simulink model "model_V1000Sim"  (R2020a)
settings: Solver=ode1  StartTime=tspan(1)  StopTime=tspan(2)  FixedStep=Ts_SimBigModel.Ts_base  RelTol=1e-3
undefined symbols (not defined in the file or in its folder): IMU1, IMU2, IMU3, mag1, mag2, SIM_SENSOR_SET
settings Model: PauseTimes=1  Creator=sl  LastModifiedBy=Administrator
settings SolverCC: AutoInsertRateTranBlk=on
settings OptimizationCC: DefaultParameterBehavior=Inlined  EnhancedBackFolding=on  PassReuseOutputArgsAs=Individual arguments  ZeroExternalMemoryAtStartup=off  ZeroInternalMemoryAtStartup=off  MaxStackSize=64  OptimizeBlockOrder=speed  DifferentSizesBufferReuse=on  OptimizationCustomize=off  EfficientTunableParamExpr=on
settings DebuggingCC: InheritedTsInSrcMsg=none  MultiTaskCondExecSysMsg=none  ParameterTunabilityLossMsg=error  UnconnectedInputMsg=none  UnconnectedOutputMsg=none  UnconnectedLineMsg=none  BusObjectLabelMismatch=error
settings HardwareCC: ProdBitPerPointer=32  ProdBitPerSizeT=32  ProdBitPerPtrDiffT=32  ProdLargestAtomicInteger=Long  ProdLargestAtomicFloat=Double  ProdWordSize=32  ProdHWDeviceType=ARM Compatible->ARM Cortex
settings ModelReferenceCC: EnableParallelModelReferenceBuilds=on  ParallelModelReferenceMATLABWorkerInit=Load Top Model
settings SFSimCC: MATLABDynamicMemAlloc=off
settings RTWCC: SystemTargetFile=ert.tlc  TemplateMakefile=ert_default_tmf  GenerateReport=on  Toolchain=GNU Tools for ARM Embedded Processors  IncludeHyperlinkInReport=on  LaunchReport=on  GenerateTraceInfo=on  GenerateTraceReport=on  GenerateTraceReportSl=on  GenerateTraceReportSf=on  GenerateTraceReportEml=on
settings CodeAppCC: ForceParamTrailComments=on  IgnoreCustomStorageClasses=off  OperatorAnnotations=on  SimulinkDataObjDesc=on  SFDataObjDesc=on  InsertBlockDesc=on
settings ERTTargetCC: InlinedParameterPlacement=NonHierarchical  ERTCustomFileTemplate=example_file_process.tlc

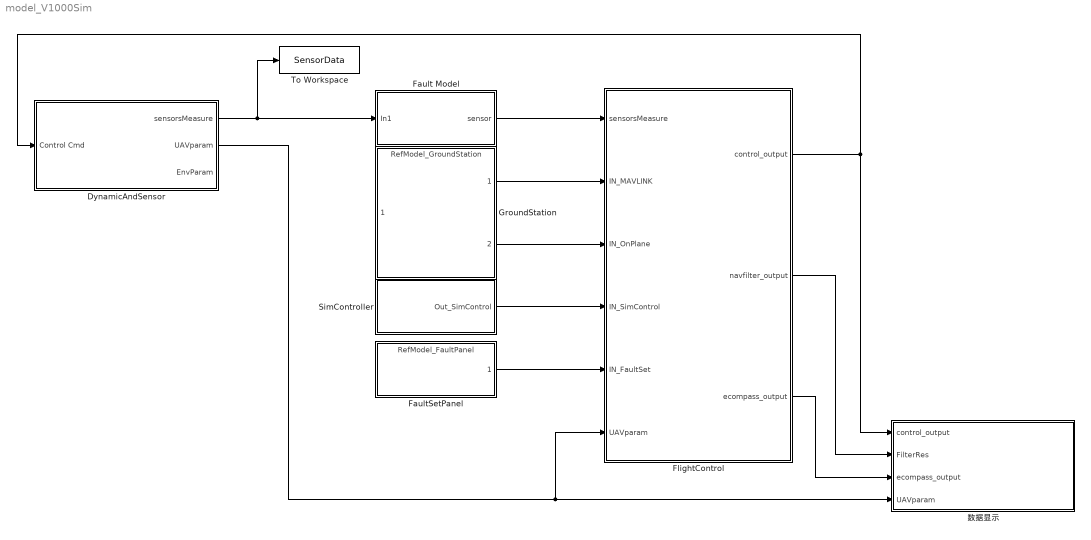
== system model_V1000Sim ==
  DynamicAndSensor : Subsystem  Variant=on
  Fault Model : Subsystem  VariantControl=SensorNoiseMode==1
  FaultSetPanel : ModelReference  ModelNameDialog=RefModel_FaultPanel  SimulationMode=Normal  ModelReferenceVersion=1.1470
  FlightControl : Subsystem
  GroundStation : ModelReference  ModelNameDialog=RefModel_GroundStation.slx  SimulationMode=Normal  CachedPortDiscreteRates=[0.04]  ModelReferenceVersion=1.3745
  SimController : Subsystem  VariantControl=SensorNoiseMode==1
  To Workspace : ToWorkspace  VariableName=SensorData  SaveFormat=Timeseries  SampleTime=-1
  数据显示 : Subsystem  Variant=on
  wires:
  FlightControl/2(navfilter_output) -> 数据显示/2(FilterRes)
  FlightControl/3(ecompass_output) -> 数据显示/3(ecompass_output)
  Fault Model/1(sensor) -> FlightControl/1(sensorsMeasure)
  DynamicAndSensor/1(sensorsMeasure) -> To Workspace/1, Fault Model/1(In1)
  DynamicAndSensor/2(UAVparam) -> FlightControl/6(UAVparam), 数据显示/4(UAVparam)
  FlightControl/1(control_output) -> DynamicAndSensor/1(Control Cmd), 数据显示/1(control_output)
  GroundStation/2 -> FlightControl/3(IN_OnPlane)
  GroundStation/1 -> FlightControl/2(IN_MAVLINK)
  SimController/1(Out_SimControl) -> FlightControl/4(IN_SimControl)
  FaultSetPanel/1 -> FlightControl/5(IN_FaultSet)

== system model_V1000Sim/DynamicAndSensor ==
  note: 1) Add Subsystem or Model blocks as valid variant choices.
      | 2) You cannot connect blocks at this level. At simulation, connectivity is automatically
      | determined, based on the active variant and port name matching.
  Control Cmd : Inport
  Flight Data : ModelReference  DisableCoverage=on  ModelNameDialog=RefModel_AeroDyn_FlightData.slx  SimulationMode=Normal  VariantControl=SimulinkRunMode == 1  ModelReferenceVersion=1.1284
  Sim Data : ModelReference  ModelNameDialog=RefModel_AeroDyn_Sim.slx  SimulationMode=Normal  VariantControl=SimulinkRunMode == 2  ModelReferenceVersion=1.1317
  sensorsMeasure : Outport
  UAVparam : Outport  Port=2
  EnvParam : Outport  Port=3  LockScale=on

== system model_V1000Sim/Fault Model ==
  In1 : Inport
  SignalFaultModel : ModelReference  Commented=through  DisableCoverage=on  ModelNameDialog=RefModel_SignalFault.slx  SimulationMode=Normal  ModelReferenceVersion=1.345
  sensor : Outport
  wires:
  In1/1 -> SignalFaultModel/1
  SignalFaultModel/1 -> sensor/1

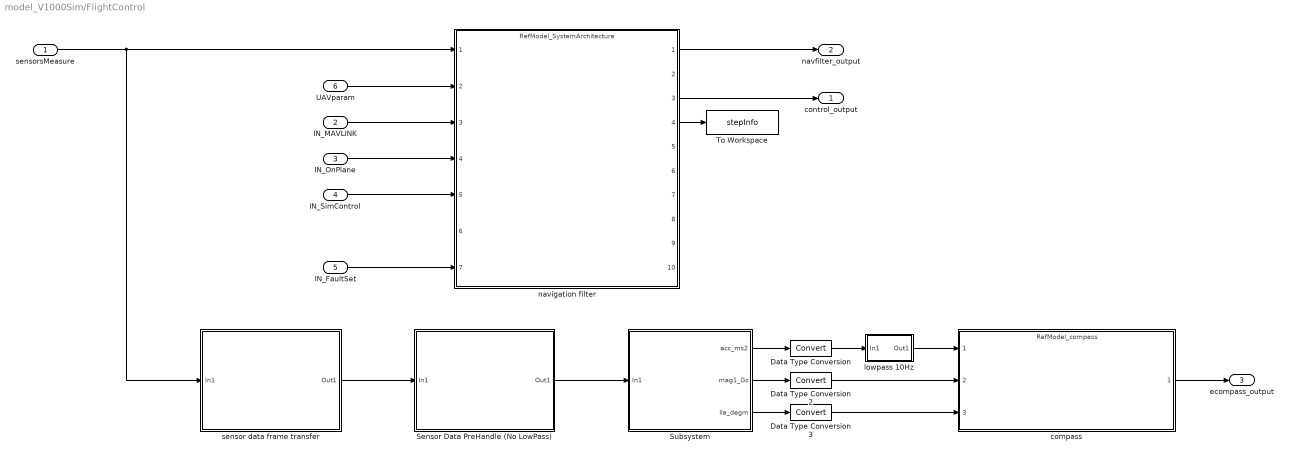
== system model_V1000Sim/FlightControl ==
  sensorsMeasure : Inport
  IN_MAVLINK : Inport  Port=2
  IN_OnPlane : Inport  Port=3
  IN_SimControl : Inport  Port=4
  IN_FaultSet : Inport  Port=5
  UAVparam : Inport  Port=6
  Data Type Conversion : DataTypeConversion
  Data Type Conversion2 : DataTypeConversion
  Data Type Conversion3 : DataTypeConversion
  Sensor Data PreHandle (No LowPass) : Subsystem
  Subsystem : Subsystem
  To Workspace : ToWorkspace  VariableName=stepInfo  SaveFormat=Timeseries  SampleTime=-1
  compass : ModelReference  ModelNameDialog=RefModel_compass.slx  SimulationMode=Normal  ModelReferenceVersion=1.16
  lowpass 10Hz : Subsystem
  navigation filter : ModelReference  ModelNameDialog=RefModel_SystemArchitecture  SimulationMode=Normal  ModelReferenceVersion=1.852
  sensor data frame transfer : Subsystem
  control_output : Outport
  navfilter_output : Outport  Port=2
  ecompass_output : Outport  Port=3
  wires:
  Subsystem/1(acc_ms2) -> Data Type Conversion/1
  Subsystem/2(mag1_Gs) -> Data Type Conversion2/1
  Subsystem/3(lla_degm) -> Data Type Conversion3/1
  Data Type Conversion2/1 -> compass/2
  Data Type Conversion3/1 -> compass/3
  Data Type Conversion/1 -> lowpass 10Hz/1(In1)
  lowpass 10Hz/1(Out1) -> compass/1
  navigation filter/1 -> navfilter_output/1
  sensorsMeasure/1 -> sensor data frame transfer/1(In1), navigation filter/1
  Sensor Data PreHandle (No LowPass)/1(Out1) -> Subsystem/1(In1)
  sensor data frame transfer/1(Out1) -> Sensor Data PreHandle (No LowPass)/1(In1)
  navigation filter/3 -> control_output/1
  UAVparam/1 -> navigation filter/2
  navigation filter/4 -> To Workspace/1
  IN_MAVLINK/1 -> navigation filter/3
  IN_OnPlane/1 -> navigation filter/4
  IN_SimControl/1 -> navigation filter/5
  compass/1 -> ecompass_output/1
  IN_FaultSet/1 -> navigation filter/7

== system model_V1000Sim/SimController ==
  10sec : Step  Time=10+33  mask(DiscretizedSource){}
      mask init:
      | %zoh
  Bus Assignment : BusAssignment  AssignedSignals=isSimOn
  Constant : Constant  Value=false
  Constant1 : Constant  Value=true
  Constant2 : Constant  Value=0  OutDataTypeStr=Bus: BUS_SIMCONTROL
  Data Type Conversion : DataTypeConversion
  Manual Switch : ManualSwitch
  Manual Switch1 : ManualSwitch
  Out_SimControl : Outport
  wires:
  Constant/1 -> Manual Switch/1
  Constant1/1 -> Manual Switch/2
  Constant2/1 -> Bus Assignment/1
  Bus Assignment/1 -> Out_SimControl/1
  Manual Switch1/1 -> Bus Assignment/2
  Manual Switch/1 -> Manual Switch1/2
  10sec/1 -> Data Type Conversion/1
  Data Type Conversion/1 -> Manual Switch1/1

== system model_V1000Sim/数据显示 ==
  note: 1) Add Subsystem or Model blocks as valid variant choices.
      | 2) You cannot connect blocks at this level. At simulation, connectivity is automatically
      | determined, based on the active variant and port name matching.
  control_output : Inport
  FilterRes : Inport  Port=2
  ecompass_output : Inport  Port=3
  UAVparam : Inport  Port=4
  Flight Data : Subsystem  VariantControl=SimulinkRunMode == 1
  Sim Data : Subsystem  VariantControl=SimulinkRunMode == 2

== system model_V1000Sim/FlightControl/Sensor Data PreHandle (No LowPass) ==
  In1 : Inport
  Bus Assignment : BusAssignment  AssignedSignals=IMU1,IMU2,IMU3,mag1,mag2
  Bus Selector : BusSelector  OutputSignals=IMU1,IMU2,IMU3
  Bus Selector1 : BusSelector  OutputSignals=mag1,mag2
  Subsystem : Subsystem
  Subsystem1 : Subsystem
  Subsystem2 : Subsystem
  Subsystem3 : Subsystem
  Subsystem4 : Subsystem
  Out1 : Outport
  wires:
  Bus Selector1/2 -> Subsystem4/1(In1)  "<mag2>"
  Bus Selector1/1 -> Subsystem3/1(In1)  "<mag1>"
  Bus Selector/3 -> Subsystem2/1(In1)  "<IMU3>"
  Bus Selector/2 -> Subsystem1/1(In1)  "<IMU2>"
  Bus Selector/1 -> Subsystem/1(In1)  "<IMU1>"
  Subsystem4/1(Out1) -> Bus Assignment/6  "mag2"
  Subsystem3/1(Out1) -> Bus Assignment/5  "mag1"
  In1/1 -> Bus Selector/1, Bus Assignment/1, Bus Selector1/1
  Bus Assignment/1 -> Out1/1
  Subsystem2/1(Out1) -> Bus Assignment/4  "IMU3"
  Subsystem1/1(Out1) -> Bus Assignment/3  "IMU2"
  Subsystem/1(Out1) -> Bus Assignment/2  "IMU1"

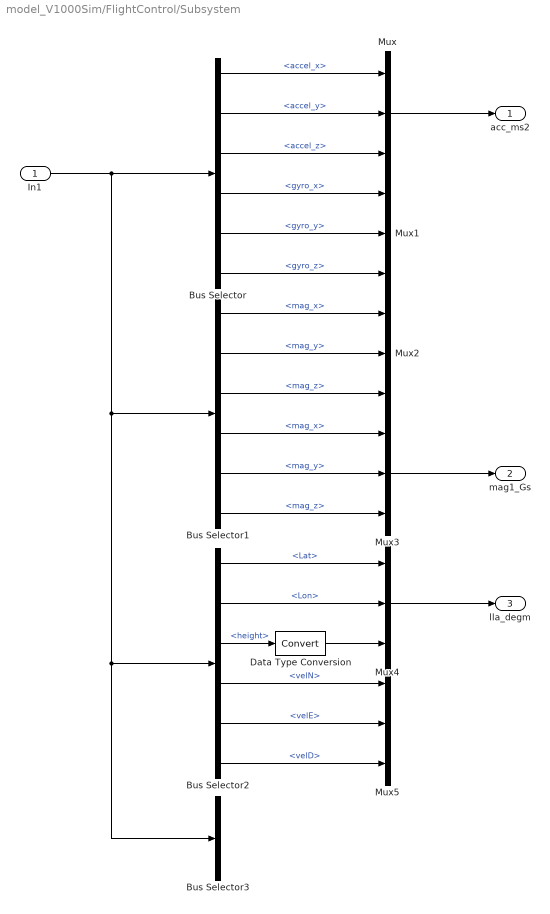
== system model_V1000Sim/FlightControl/Subsystem ==
  In1 : Inport
  Bus Selector : BusSelector  OutputSignals=IMU1.accel_x,IMU1.accel_y,IMU1.accel_z,IMU1.gyro_x,IMU1.gyro_y,IMU1.gyro_z
  Bus Selector1 : BusSelector  OutputSignals=mag1.mag_x,mag1.mag_y,mag1.mag_z,mag2.mag_x,mag2.mag_y,mag2.mag_z
  Bus Selector2 : BusSelector  OutputSignals=ublox1.Lat,ublox1.Lon,ublox1.height,ublox1.velN,ublox1.velE,ublox1.velD
  Bus Selector3 : BusSelector  OutputSignals=baro1.alt_baro,radar1.Range
  Data Type Conversion : DataTypeConversion
  Mux{,1..5} (6 alike) : Mux  Inputs=3
  acc_ms2 : Outport
  mag1_Gs : Outport  Port=2
  lla_degm : Outport  Port=3
  wires:
  In1/1 -> Bus Selector3/1, Bus Selector2/1, Bus Selector1/1, Bus Selector/1
  Bus Selector/1 -> Mux/1  "<accel_x>"
  Bus Selector/2 -> Mux/2  "<accel_y>"
  Bus Selector/3 -> Mux/3  "<accel_z>"
  Bus Selector/4 -> Mux1/1  "<gyro_x>"
  Bus Selector/5 -> Mux1/2  "<gyro_y>"
  Bus Selector/6 -> Mux1/3  "<gyro_z>"
  Mux/1 -> acc_ms2/1
  Bus Selector1/1 -> Mux2/1  "<mag_x>"
  Bus Selector1/2 -> Mux2/2  "<mag_y>"
  Bus Selector1/3 -> Mux2/3  "<mag_z>"
  Bus Selector1/4 -> Mux3/1  "<mag_x>"
  Bus Selector1/5 -> Mux3/2  "<mag_y>"
  Bus Selector1/6 -> Mux3/3  "<mag_z>"
  Bus Selector2/6 -> Mux5/3  "<velD>"
  Bus Selector2/5 -> Mux5/2  "<velE>"
  Bus Selector2/4 -> Mux5/1  "<velN>"
  Bus Selector2/3 -> Data Type Conversion/1  "<height>"
  Bus Selector2/2 -> Mux4/2  "<Lon>"
  Bus Selector2/1 -> Mux4/1  "<Lat>"
  Mux4/1 -> lla_degm/1
  Data Type Conversion/1 -> Mux4/3
  Mux3/1 -> mag1_Gs/1

== system model_V1000Sim/FlightControl/lowpass 10Hz ==
  In1 : Inport
  Demux : Demux  Outputs=3
  Mux : Mux  Inputs=3
  Mux1 : Mux  Inputs=2
  Mux2 : Mux  Inputs=2
  Mux3 : Mux  Inputs=2
  Scope : Scope  NumInputPorts=3
  Transfer Fcn : TransferFcn  Denominator=[.1 1]
  Transfer Fcn1 : TransferFcn  Denominator=[.1 1]
  Transfer Fcn2 : TransferFcn  Denominator=[.1 1]
  Out1 : Outport
  wires:
  In1/1 -> Demux/1
  Demux/1 -> Mux1/1, Transfer Fcn/1  "orignial x"
  Demux/2 -> Mux2/1, Transfer Fcn1/1  "orignial y"
  Mux/1 -> Out1/1
  Transfer Fcn1/1 -> Mux2/2, Mux/2  "filter y"
  Transfer Fcn2/1 -> Mux3/2, Mux/3  "filter z"
  Transfer Fcn/1 -> Mux1/2, Mux/1  "filter x"
  Demux/3 -> Mux3/1, Transfer Fcn2/1  "orignial z"
  Mux1/1 -> Scope/1  "ax"
  Mux2/1 -> Scope/2  "ay"
  Mux3/1 -> Scope/3  "az"

== system model_V1000Sim/FlightControl/sensor data frame transfer ==
  In1 : Inport
  Bus Assignment : BusAssignment  AssignedSignals=IMU1,IMU2,IMU3,mag1,mag2
  Bus Selector : BusSelector  OutputSignals=IMU1,IMU2,IMU3
  Bus Selector1 : BusSelector  OutputSignals=mag1,mag2
  SensorFrame to BodyFrame : Subsystem
  SensorFrame to BodyFrame1 : Subsystem
  SensorFrame to BodyFrame2 : Subsystem
  SensorFrame to BodyFrame3 : Subsystem
  SensorFrame to BodyFrame4 : Subsystem
  Out1 : Outport
  wires:
  Bus Selector/1 -> SensorFrame to BodyFrame/1(In1)  "<IMU1>"
  Bus Selector/2 -> SensorFrame to BodyFrame1/1(In1)  "<IMU2>"
  Bus Selector/3 -> SensorFrame to BodyFrame2/1(In1)  "<IMU3>"
  SensorFrame to BodyFrame/1(Out1) -> Bus Assignment/2  "IMU1"
  SensorFrame to BodyFrame1/1(Out1) -> Bus Assignment/3  "IMU2"
  SensorFrame to BodyFrame2/1(Out1) -> Bus Assignment/4  "IMU3"
  Bus Assignment/1 -> Out1/1
  In1/1 -> Bus Selector1/1, Bus Assignment/1, Bus Selector/1
  Bus Selector1/1 -> SensorFrame to BodyFrame3/1(In1)  "<mag1>"
  Bus Selector1/2 -> SensorFrame to BodyFrame4/1(In1)  "<mag2>"
  SensorFrame to BodyFrame3/1(Out1) -> Bus Assignment/5  "mag1"
  SensorFrame to BodyFrame4/1(Out1) -> Bus Assignment/6  "mag2"

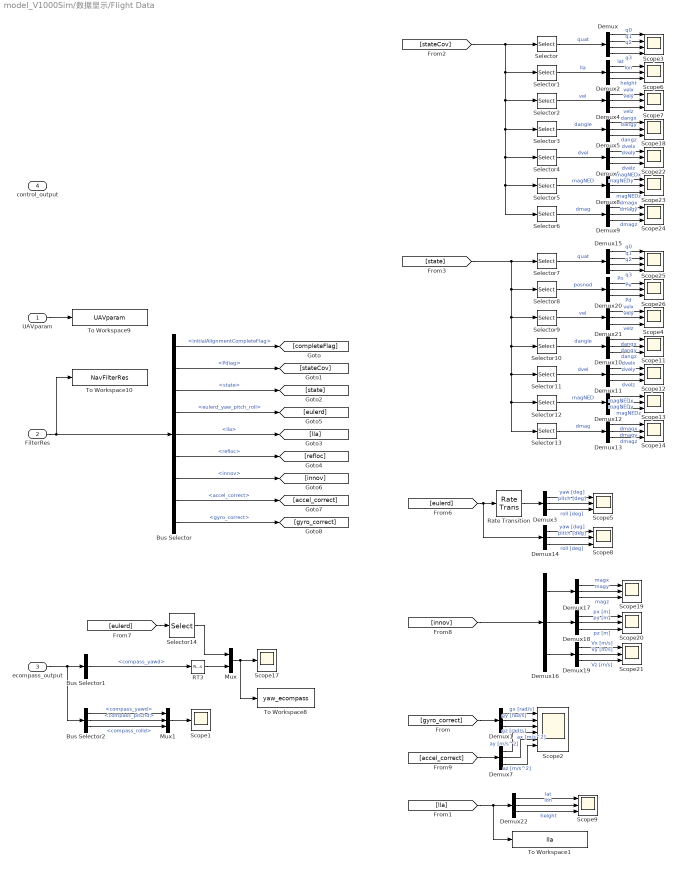
== system model_V1000Sim/数据显示/Flight Data ==
  UAVparam : Inport
  FilterRes : Inport  Port=2
  ecompass_output : Inport  Port=3
  control_output : Inport  Port=4
  Bus Selector : BusSelector  OutputSignals=initialAlignmentCompleteFlag,Pdiag,state,eulerd_yaw_pitch_roll,lla,refloc,innov,accel_correct,gyro_correct
  Bus Selector1 : BusSelector  OutputSignals=compass_yawd
  Bus Selector2 : BusSelector  OutputSignals=compass_yawd,compass_pitchd,compass_rolld
  Demux : Demux
  Demux{1..14,16..22} (21 alike) : Demux  Outputs=3
  Demux15 : Demux
  Mux : Mux  Inputs=2
  Mux1 : Mux  Inputs=3
  RT3 : RateTransition
  Rate Transition : RateTransition  OutPortSampleTime=0.012
  Scope1 : Scope
  Scope{4..9,11..14,18..24,26} (18 alike) : Scope  NumInputPorts=3
  Scope17 : Scope
  Scope2 : Scope  NumInputPorts=6
  Scope25 : Scope  NumInputPorts=4
  Scope3 : Scope  NumInputPorts=4
  Selector : Selector  InputPortWidth=nStateMARG  IndexOptions=Index vector (dialog)  Indices=[1:4]  OutputSizes=1
  Selector1 : Selector  InputPortWidth=nStateMARG  IndexOptions=Index vector (dialog)  Indices=[5:7]  OutputSizes=1
  Selector10 : Selector  InputPortWidth=nStateMARG  IndexOptions=Index vector (dialog)  Indices=[11:13]  OutputSizes=1
  Selector11 : Selector  InputPortWidth=nStateMARG  IndexOptions=Index vector (dialog)  Indices=[14:16]  OutputSizes=1
  Selector12 : Selector  InputPortWidth=nStateMARG  IndexOptions=Index vector (dialog)  Indices=[17:19]  OutputSizes=1
  Selector13 : Selector  InputPortWidth=nStateMARG  IndexOptions=Index vector (dialog)  Indices=[20:22]  OutputSizes=1
  Selector14 : Selector  InputPortWidth=3  IndexOptions=Index vector (dialog)  Indices=1  OutputSizes=1
  Selector2 : Selector  InputPortWidth=nStateMARG  IndexOptions=Index vector (dialog)  Indices=[8:10]  OutputSizes=1
  Selector3 : Selector  InputPortWidth=nStateMARG  IndexOptions=Index vector (dialog)  Indices=[11:13]  OutputSizes=1
  Selector4 : Selector  InputPortWidth=nStateMARG  IndexOptions=Index vector (dialog)  Indices=[14:16]  OutputSizes=1
  Selector5 : Selector  InputPortWidth=nStateMARG  IndexOptions=Index vector (dialog)  Indices=[17:19]  OutputSizes=1
  Selector6 : Selector  InputPortWidth=nStateMARG  IndexOptions=Index vector (dialog)  Indices=[20:22]  OutputSizes=1
  Selector7 : Selector  InputPortWidth=nStateMARG  IndexOptions=Index vector (dialog)  Indices=[1:4]  OutputSizes=1
  Selector8 : Selector  InputPortWidth=nStateMARG  IndexOptions=Index vector (dialog)  Indices=[5:7]  OutputSizes=1
  Selector9 : Selector  InputPortWidth=nStateMARG  IndexOptions=Index vector (dialog)  Indices=[8:10]  OutputSizes=1
  To Workspace1 : ToWorkspace  VariableName=lla  SaveFormat=Timeseries  SampleTime=-1
  To Workspace10 : ToWorkspace  VariableName=NavFilterRes  SaveFormat=Timeseries  SampleTime=-1
  To Workspace8 : ToWorkspace  VariableName=yaw_ecompass  SaveFormat=Timeseries  SampleTime=-1
  To Workspace9 : ToWorkspace  VariableName=UAVparam  SaveFormat=Timeseries  SampleTime=-1
  wires:
  Demux13/1 -> Scope14/1  "dmagx"
  Demux16/2 -> Demux18/1
  Demux21/3 -> Scope4/3  "velz"
  Demux12/1 -> Scope13/1  "magNEDx"
  Selector14/1 -> Mux/1
  Demux10/1 -> Scope11/1  "dangx"
  Demux12/2 -> Scope13/2  "magNEDy"
  Selector10/1 -> Demux10/1  "dangle"
  Demux15/4 -> Scope25/4  "q3"
  Demux19/2 -> Scope21/2  "Vy [m/s]"
  Selector1/1 -> Demux2/1  "lla"
  Demux3/2 -> Scope5/2  "pitch [deg]"
  Demux18/1 -> Scope20/1  "px [m]"
  [state] -> Selector8/1, Selector11/1, Selector12/1, Selector13/1, Selector10/1, Selector9/1, Selector7/1
  Demux5/2 -> Scope18/2  "dangy"
  Selector12/1 -> Demux12/1  "magNED"
  Selector13/1 -> Demux13/1  "dmag"
  Demux17/2 -> Scope19/2  "magy"
  Demux11/1 -> Scope12/1  "dvelx"
  [innov] -> Demux16/1
  Demux18/2 -> Scope20/2  "py [m]"
  Demux11/2 -> Scope12/2  "dvely"
  Demux15/3 -> Scope25/3  "q2"
  Demux16/3 -> Demux19/1
  Demux19/1 -> Scope21/1  "Vx [m/s]"
  Demux6/3 -> Scope22/3  "dvelz"
  Mux/1 -> To Workspace8/1, Scope17/1
  Demux15/2 -> Scope25/2  "q1"
  Bus Selector1/1 -> RT3/1  "<compass_yawd>"
  [eulerd] -> Demux14/1, Rate Transition/1
  [eulerd] -> Selector14/1
  Demux17/3 -> Scope19/3  "magz"
  Demux10/3 -> Scope11/3  "dangz"
  Demux21/1 -> Scope4/1  "velx"
  Demux/2 -> Scope3/2  "q1"
  Demux16/1 -> Demux17/1
  Demux/1 -> Scope3/1  "q0"
  [stateCov] -> Selector/1, Selector3/1, Selector4/1, Selector5/1, Selector6/1, Selector2/1, Selector1/1
  Demux9/2 -> Scope24/2  "dmagy"
  Demux/3 -> Scope3/3  "q2"
  Selector2/1 -> Demux4/1  "vel"
  Demux19/3 -> Scope21/3  "Vz [m/s]"
  Demux13/2 -> Scope14/2  "dmagy"
  Selector6/1 -> Demux9/1  "dmag"
  Demux17/1 -> Scope19/1  "magx"
  RT3/1 -> Mux/2
  Demux/4 -> Scope3/4  "q3"
  Demux2/1 -> Scope6/1  "lat"
  Demux2/3 -> Scope6/3  "height"
  Selector/1 -> Demux/1  "quat"
  Demux5/3 -> Scope18/3  "dangz"
  Demux4/3 -> Scope7/3  "velz"
  Demux10/2 -> Scope11/2  "dangy"
  Demux4/2 -> Scope7/2  "vely"
  Demux8/2 -> Scope23/2  "magNEDy"
  Demux18/3 -> Scope20/3  "pz [m]"
  Selector3/1 -> Demux5/1  "dangle"
  Demux2/2 -> Scope6/2  "lon"
  Selector5/1 -> Demux8/1  "magNED"
  Demux8/1 -> Scope23/1  "magNEDx"
  Demux6/2 -> Scope22/2  "dvely"
  Demux9/3 -> Scope24/3  "dmagz"
  Demux12/3 -> Scope13/3  "magNEDz"
  Demux3/3 -> Scope5/3  "roll [deg]"
  Demux21/2 -> Scope4/2  "vely"
  Demux8/3 -> Scope23/3  "magNEDz"
  Selector11/1 -> Demux11/1  "dvel"
  Selector9/1 -> Demux21/1  "vel"
  Demux20/3 -> Scope26/3  "Pd"
  Selector7/1 -> Demux15/1  "quat"
  Demux13/3 -> Scope14/3  "dmagz"
  Demux20/2 -> Scope26/2  "Pe"
  Selector4/1 -> Demux6/1  "dvel"
  Selector8/1 -> Demux20/1  "posned"
  Demux3/1 -> Scope5/1  "yaw [deg]"
  Demux11/3 -> Scope12/3  "dvelz"
  Demux15/1 -> Scope25/1  "q0"
  Demux20/1 -> Scope26/1  "Pn"
  Demux5/1 -> Scope18/1  "dangx"
  Demux6/1 -> Scope22/1  "dvelx"
  Demux4/1 -> Scope7/1  "velx"
  Demux9/1 -> Scope24/1  "dmagx"
  FilterRes/1 -> To Workspace10/1, Bus Selector/1
  Bus Selector/4 -> [eulerd]  "<eulerd_yaw_pitch_roll>"
  Bus Selector/3 -> [state]  "<state>"
  Bus Selector/5 -> [lla]  "<lla>"
  Bus Selector/2 -> [stateCov]  "<Pdiag>"
  Bus Selector/6 -> [refloc]  "<refloc>"
  Bus Selector/1 -> [completeFlag]  "<initialAlignmentCompleteFlag>"
  Bus Selector/7 -> [innov]  "<innov>"
  ecompass_output/1 -> Bus Selector2/1, Bus Selector1/1
  Bus Selector/8 -> [accel_correct]  "<accel_correct>"
  Bus Selector/9 -> [gyro_correct]  "<gyro_correct>"
  Bus Selector2/1 -> Mux1/1  "<compass_yawd>"
  Bus Selector2/2 -> Mux1/2  "<compass_pitchd>"
  Bus Selector2/3 -> Mux1/3  "<compass_rolld>"
  Mux1/1 -> Scope1/1
  [gyro_correct] -> Demux1/1
  [accel_correct] -> Demux7/1
  Demux1/1 -> Scope2/1  "gx [rad/s]"
  Demux1/2 -> Scope2/2  "gy [rad/s]"
  Demux1/3 -> Scope2/3  "gz [rad/s]"
  Demux7/1 -> Scope2/4  "ax [m/s^2]"
  Demux7/2 -> Scope2/5  "ay [m/s^2]"
  Demux7/3 -> Scope2/6  "az [m/s^2]"
  UAVparam/1 -> To Workspace9/1
  Rate Transition/1 -> Demux3/1
  Demux14/1 -> Scope8/1  "yaw [deg]"
  Demux14/3 -> Scope8/3  "roll [deg]"
  Demux14/2 -> Scope8/2  "pitch [deg]"
  Demux22/1 -> Scope9/1  "lat"
  Demux22/2 -> Scope9/2  "lon"
  Demux22/3 -> Scope9/3  "height"
  [lla] -> To Workspace1/1, Demux22/1

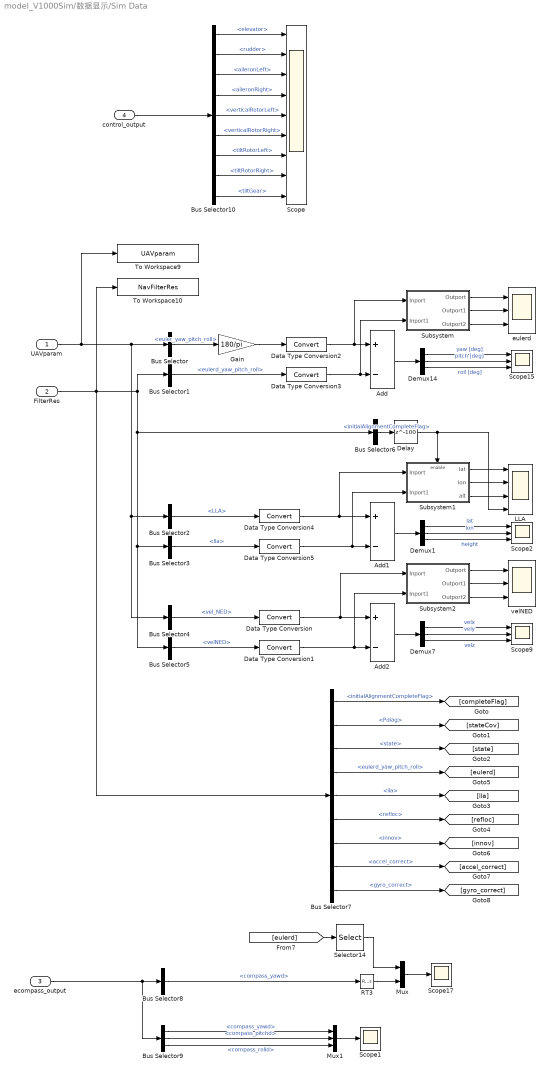
== system model_V1000Sim/数据显示/Sim Data ==
  UAVparam : Inport
  FilterRes : Inport  Port=2
  ecompass_output : Inport  Port=3
  control_output : Inport  Port=4
  Add : Sum  Inputs=+-
  Add1 : Sum  Inputs=+-
  Add2 : Sum  Inputs=+-
  Bus Selector : BusSelector  OutputSignals=euler_yaw_pitch_roll
  Bus Selector1 : BusSelector  OutputSignals=eulerd_yaw_pitch_roll
  Bus Selector10 : BusSelector  OutputSignals=elevator,rudder,aileronLeft,aileronRight,verticalRotorLeft,verticalRotorRight,tiltRotorLeft,tiltRotorRight,tiltGear
  Bus Selector2 : BusSelector  OutputSignals=LLA
  Bus Selector3 : BusSelector  OutputSignals=lla
  Bus Selector4 : BusSelector  OutputSignals=vel_NED
  Bus Selector5 : BusSelector  OutputSignals=velNED
  Bus Selector6 : BusSelector  OutputSignals=initialAlignmentCompleteFlag
  Bus Selector7 : BusSelector  OutputSignals=initialAlignmentCompleteFlag,Pdiag,state,eulerd_yaw_pitch_roll,lla,refloc,innov,accel_correct,gyro_correct
  Bus Selector8 : BusSelector  OutputSignals=compass_yawd
  Bus Selector9 : BusSelector  OutputSignals=compass_yawd,compass_pitchd,compass_rolld
  Data Type Conversion{,1..5} (6 alike) : DataTypeConversion
  Delay : Delay  DelayLength=100
  Demux1 : Demux  Outputs=3
  Demux14 : Demux  Outputs=3
  Demux7 : Demux  Outputs=3
  Gain : Gain  Gain=180/pi
  LLA : Scope  NumInputPorts=4
  Mux : Mux  Inputs=2
  Mux1 : Mux  Inputs=3
  RT3 : RateTransition
  Scope : Scope  NumInputPorts=9
  Scope1 : Scope
  Scope15 : Scope  NumInputPorts=3
  Scope17 : Scope
  Scope2 : Scope  NumInputPorts=3
  Scope9 : Scope  NumInputPorts=3
  Selector14 : Selector  InputPortWidth=3  IndexOptions=Index vector (dialog)  Indices=1  OutputSizes=1
  Subsystem : Subsystem
  Subsystem1 : Subsystem
  Subsystem2 : Subsystem
  To Workspace10 : ToWorkspace  VariableName=NavFilterRes  SaveFormat=Timeseries  SampleTime=-1
  To Workspace9 : ToWorkspace  VariableName=UAVparam  SaveFormat=Timeseries  SampleTime=-1
  eulerd : Scope  NumInputPorts=3
  velNED : Scope  NumInputPorts=3
  wires:
  Demux14/3 -> Scope15/3  "roll [deg]"
  Bus Selector4/1 -> Data Type Conversion/1  "<vel_NED>"
  Demux14/2 -> Scope15/2  "pitch [deg]"
  Bus Selector2/1 -> Data Type Conversion4/1  "<LLA>"
  Demux1/3 -> Scope2/3  "height"
  Gain/1 -> Data Type Conversion2/1
  Bus Selector3/1 -> Data Type Conversion5/1  "<lla>"
  Demux1/1 -> Scope2/1  "lat"
  Demux7/3 -> Scope9/3  "velz"
  Subsystem2/3(Outport2) -> velNED/3
  Bus Selector1/1 -> Data Type Conversion3/1  "<eulerd_yaw_pitch_roll>"
  Subsystem2/2(Outport1) -> velNED/2
  Demux7/1 -> Scope9/1  "velx"
  Demux14/1 -> Scope15/1  "yaw [deg]"
  Subsystem1/2(lon) -> LLA/2
  Add2/1 -> Demux7/1
  Add1/1 -> Demux1/1
  Subsystem1/1(lat) -> LLA/1
  Subsystem/3(Outport2) -> eulerd/3
  Demux1/2 -> Scope2/2  "lon"
  Add/1 -> Demux14/1
  Subsystem2/1(Outport) -> velNED/1
  Bus Selector/1 -> Gain/1  "<euler_yaw_pitch_roll>"
  Demux7/2 -> Scope9/2  "vely"
  Subsystem1/3(alt) -> LLA/3
  Subsystem/2(Outport1) -> eulerd/2
  Subsystem/1(Outport) -> eulerd/1
  Bus Selector5/1 -> Data Type Conversion1/1  "<velNED>"
  UAVparam/1 -> To Workspace9/1, Bus Selector2/1, Bus Selector4/1, Bus Selector/1
  Bus Selector6/1 -> Delay/1  "<initialAlignmentCompleteFlag>"
  Delay/1 -> LLA/4, Subsystem1/Enable
  FilterRes/1 -> Bus Selector7/1, Bus Selector6/1, Bus Selector3/1, Bus Selector5/1, Bus Selector1/1, To Workspace10/1
  Mux1/1 -> Scope1/1
  Bus Selector9/3 -> Mux1/3  "<compass_rolld>"
  Bus Selector9/1 -> Mux1/1  "<compass_yawd>"
  Bus Selector9/2 -> Mux1/2  "<compass_pitchd>"
  [eulerd] -> Selector14/1
  Mux/1 -> Scope17/1
  Bus Selector8/1 -> RT3/1  "<compass_yawd>"
  RT3/1 -> Mux/2
  ecompass_output/1 -> Bus Selector9/1, Bus Selector8/1
  Selector14/1 -> Mux/1
  Bus Selector7/8 -> [accel_correct]  "<accel_correct>"
  Bus Selector7/3 -> [state]  "<state>"
  Bus Selector7/9 -> [gyro_correct]  "<gyro_correct>"
  Bus Selector7/7 -> [innov]  "<innov>"
  Bus Selector7/2 -> [stateCov]  "<Pdiag>"
  Bus Selector7/6 -> [refloc]  "<refloc>"
  Bus Selector7/1 -> [completeFlag]  "<initialAlignmentCompleteFlag>"
  Bus Selector7/5 -> [lla]  "<lla>"
  Bus Selector7/4 -> [eulerd]  "<eulerd_yaw_pitch_roll>"
  Data Type Conversion/1 -> Subsystem2/1(Inport), Add2/1
  Data Type Conversion1/1 -> Subsystem2/2(Inport1), Add2/2
  Data Type Conversion2/1 -> Subsystem/1(Inport), Add/1
  Data Type Conversion3/1 -> Subsystem/2(Inport1), Add/2
  Data Type Conversion4/1 -> Subsystem1/1(Inport), Add1/1
  Data Type Conversion5/1 -> Subsystem1/2(Inport1), Add1/2
  Bus Selector10/8 -> Scope/8  "<tiltRotorRight>"
  Bus Selector10/6 -> Scope/6  "<verticalRotorRight>"
  Bus Selector10/1 -> Scope/1  "<elevator>"
  Bus Selector10/7 -> Scope/7  "<tiltRotorLeft>"
  Bus Selector10/2 -> Scope/2  "<rudder>"
  Bus Selector10/5 -> Scope/5  "<verticalRotorLeft>"
  Bus Selector10/3 -> Scope/3  "<aileronLeft>"
  Bus Selector10/4 -> Scope/4  "<aileronRight>"
  Bus Selector10/9 -> Scope/9  "<tiltGear>"
  control_output/1 -> Bus Selector10/1

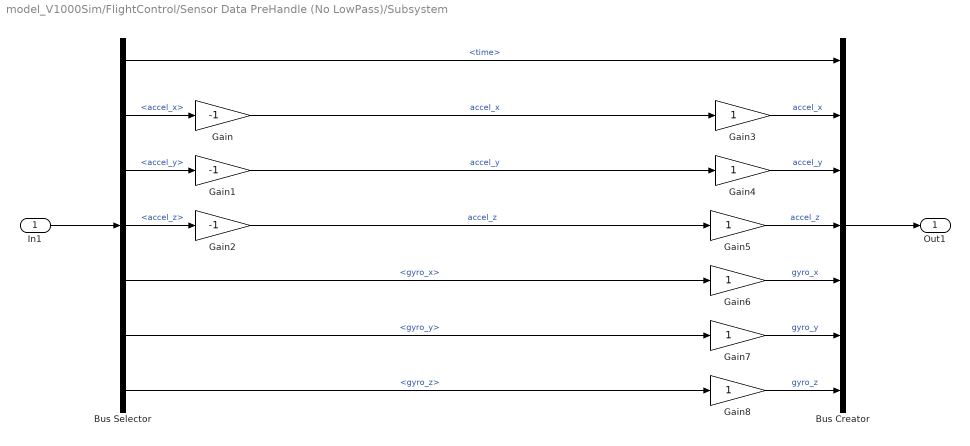
== system model_V1000Sim/FlightControl/Sensor Data PreHandle (No LowPass)/Subsystem ==
  In1 : Inport
  Bus Creator : BusCreator  Inputs=7
  Bus Selector : BusSelector  OutputSignals=time,accel_x,accel_y,accel_z,gyro_x,gyro_y,gyro_z
  Gain : Gain  Gain=-1
  Gain1 : Gain  Gain=-1
  Gain2 : Gain  Gain=-1
  Gain{3..8} (6 alike) : Gain
  Out1 : Outport
  wires:
  Gain8/1 -> Bus Creator/7  "gyro_z"
  Gain7/1 -> Bus Creator/6  "gyro_y"
  Gain6/1 -> Bus Creator/5  "gyro_x"
  Gain5/1 -> Bus Creator/4  "accel_z"
  Gain4/1 -> Bus Creator/3  "accel_y"
  Gain3/1 -> Bus Creator/2  "accel_x"
  Bus Selector/7 -> Gain8/1  "<gyro_z>"
  Bus Selector/6 -> Gain7/1  "<gyro_y>"
  Bus Selector/5 -> Gain6/1  "<gyro_x>"
  Gain2/1 -> Gain5/1  "accel_z"
  Gain1/1 -> Gain4/1  "accel_y"
  Gain/1 -> Gain3/1  "accel_x"
  Bus Selector/1 -> Bus Creator/1  "<time>"
  Bus Selector/4 -> Gain2/1  "<accel_z>"
  Bus Selector/3 -> Gain1/1  "<accel_y>"
  Bus Selector/2 -> Gain/1  "<accel_x>"
  Bus Creator/1 -> Out1/1
  In1/1 -> Bus Selector/1

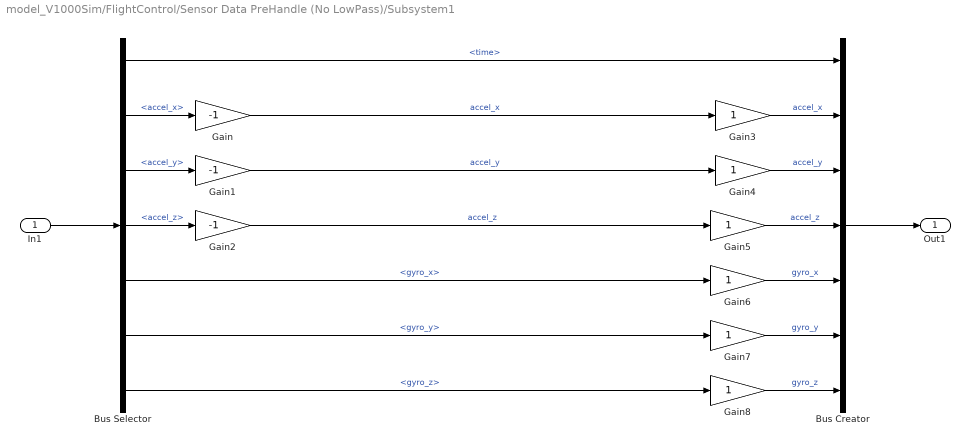
== system model_V1000Sim/FlightControl/Sensor Data PreHandle (No LowPass)/Subsystem1 ==
  In1 : Inport
  Bus Creator : BusCreator  Inputs=7
  Bus Selector : BusSelector  OutputSignals=time,accel_x,accel_y,accel_z,gyro_x,gyro_y,gyro_z
  Gain : Gain  Gain=-1
  Gain1 : Gain  Gain=-1
  Gain2 : Gain  Gain=-1
  Gain{3..8} (6 alike) : Gain
  Out1 : Outport
  wires:
  In1/1 -> Bus Selector/1
  Bus Creator/1 -> Out1/1
  Bus Selector/2 -> Gain/1  "<accel_x>"
  Bus Selector/3 -> Gain1/1  "<accel_y>"
  Bus Selector/4 -> Gain2/1  "<accel_z>"
  Bus Selector/1 -> Bus Creator/1  "<time>"
  Gain/1 -> Gain3/1  "accel_x"
  Gain1/1 -> Gain4/1  "accel_y"
  Gain2/1 -> Gain5/1  "accel_z"
  Bus Selector/5 -> Gain6/1  "<gyro_x>"
  Bus Selector/6 -> Gain7/1  "<gyro_y>"
  Bus Selector/7 -> Gain8/1  "<gyro_z>"
  Gain3/1 -> Bus Creator/2  "accel_x"
  Gain4/1 -> Bus Creator/3  "accel_y"
  Gain5/1 -> Bus Creator/4  "accel_z"
  Gain6/1 -> Bus Creator/5  "gyro_x"
  Gain7/1 -> Bus Creator/6  "gyro_y"
  Gain8/1 -> Bus Creator/7  "gyro_z"

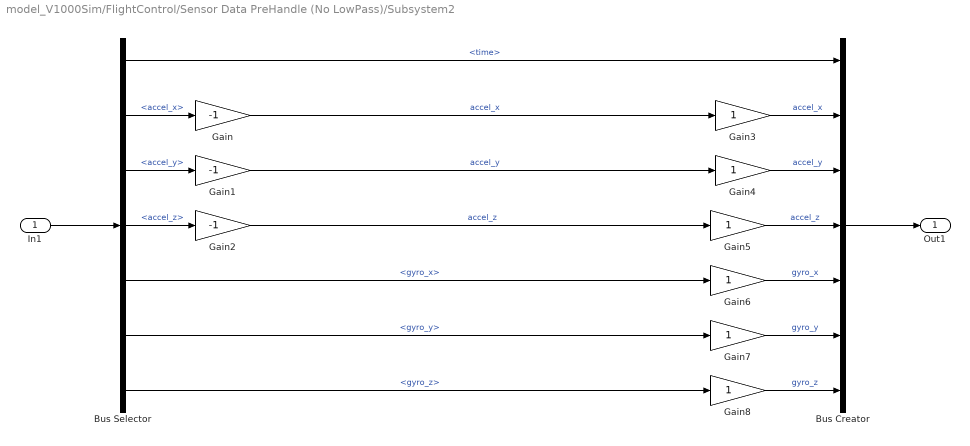
== system model_V1000Sim/FlightControl/Sensor Data PreHandle (No LowPass)/Subsystem2 ==
  In1 : Inport
  Bus Creator : BusCreator  Inputs=7
  Bus Selector : BusSelector  OutputSignals=time,accel_x,accel_y,accel_z,gyro_x,gyro_y,gyro_z
  Gain : Gain  Gain=-1
  Gain1 : Gain  Gain=-1
  Gain2 : Gain  Gain=-1
  Gain{3..8} (6 alike) : Gain
  Out1 : Outport
  wires:
  Gain8/1 -> Bus Creator/7  "gyro_z"
  Gain7/1 -> Bus Creator/6  "gyro_y"
  Gain6/1 -> Bus Creator/5  "gyro_x"
  Gain5/1 -> Bus Creator/4  "accel_z"
  Gain4/1 -> Bus Creator/3  "accel_y"
  Gain3/1 -> Bus Creator/2  "accel_x"
  Bus Selector/7 -> Gain8/1  "<gyro_z>"
  Bus Selector/6 -> Gain7/1  "<gyro_y>"
  Bus Selector/5 -> Gain6/1  "<gyro_x>"
  Gain2/1 -> Gain5/1  "accel_z"
  Gain1/1 -> Gain4/1  "accel_y"
  Gain/1 -> Gain3/1  "accel_x"
  Bus Selector/1 -> Bus Creator/1  "<time>"
  Bus Selector/4 -> Gain2/1  "<accel_z>"
  Bus Selector/3 -> Gain1/1  "<accel_y>"
  Bus Selector/2 -> Gain/1  "<accel_x>"
  Bus Creator/1 -> Out1/1
  In1/1 -> Bus Selector/1

== system model_V1000Sim/FlightControl/Sensor Data PreHandle (No LowPass)/Subsystem3 ==
  In1 : Inport
  Bus Creator : BusCreator  Inputs=4
  Bus Selector : BusSelector  OutputSignals=time,mag_x,mag_y,mag_z
  Gs to uT1 : Gain  Gain=100
  Gs to uT2 : Gain  Gain=100
  Gs to uT3 : Gain  Gain=100
  Out1 : Outport
  wires:
  Bus Selector/4 -> Gs to uT3/1  "<mag_z>"
  Bus Selector/3 -> Gs to uT2/1  "<mag_y>"
  Bus Selector/2 -> Gs to uT1/1  "<mag_x>"
  Gs to uT3/1 -> Bus Creator/4  "mag_z"
  Gs to uT2/1 -> Bus Creator/3  "mag_y"
  Gs to uT1/1 -> Bus Creator/2  "mag_x"
  In1/1 -> Bus Selector/1
  Bus Creator/1 -> Out1/1
  Bus Selector/1 -> Bus Creator/1  "<time>"

== system model_V1000Sim/FlightControl/Sensor Data PreHandle (No LowPass)/Subsystem4 ==
  In1 : Inport
  Bus Creator : BusCreator  Inputs=4
  Bus Selector : BusSelector  OutputSignals=time,mag_x,mag_y,mag_z
  Gs to uT1 : Gain  Gain=100
  Gs to uT2 : Gain  Gain=100
  Gs to uT3 : Gain  Gain=100
  Out1 : Outport
  wires:
  Bus Selector/1 -> Bus Creator/1  "<time>"
  Bus Creator/1 -> Out1/1
  In1/1 -> Bus Selector/1
  Gs to uT1/1 -> Bus Creator/2  "mag_x"
  Gs to uT2/1 -> Bus Creator/3  "mag_y"
  Gs to uT3/1 -> Bus Creator/4  "mag_z"
  Bus Selector/2 -> Gs to uT1/1  "<mag_x>"
  Bus Selector/3 -> Gs to uT2/1  "<mag_y>"
  Bus Selector/4 -> Gs to uT3/1  "<mag_z>"

== system model_V1000Sim/FlightControl/sensor data frame transfer/SensorFrame to BodyFrame ==
  In1 : Inport
  Bus Creator : BusCreator  Inputs=7
  Bus Selector : BusSelector  OutputSignals=time,accel_x,accel_y,accel_z,gyro_x,gyro_y,gyro_z
  Frame Transfer : Subsystem
  Frame Transfer1 : Subsystem
  Out1 : Outport
  wires:
  Bus Selector/1 -> Bus Creator/1  "<time>"
  Bus Creator/1 -> Out1/1
  In1/1 -> Bus Selector/1
  Bus Selector/2 -> Frame Transfer/1(In1)  "<accel_x>"
  Bus Selector/3 -> Frame Transfer/2(In2)  "<accel_y>"
  Bus Selector/4 -> Frame Transfer/3(In3)  "<accel_z>"
  Frame Transfer/1(Out1) -> Bus Creator/2  "accel_x"
  Frame Transfer/2(Out2) -> Bus Creator/3  "accel_y"
  Frame Transfer/3(Out3) -> Bus Creator/4  "accel_z"
  Bus Selector/5 -> Frame Transfer1/1(In1)  "<gyro_x>"
  Bus Selector/6 -> Frame Transfer1/2(In2)  "<gyro_y>"
  Bus Selector/7 -> Frame Transfer1/3(In3)  "<gyro_z>"
  Frame Transfer1/1(Out1) -> Bus Creator/5  "gyro_x"
  Frame Transfer1/2(Out2) -> Bus Creator/6  "gyro_y"
  Frame Transfer1/3(Out3) -> Bus Creator/7  "gyro_z"

== system model_V1000Sim/FlightControl/sensor data frame transfer/SensorFrame to BodyFrame1 ==
  In1 : Inport
  Bus Creator : BusCreator  Inputs=7
  Bus Selector : BusSelector  OutputSignals=time,accel_x,accel_y,accel_z,gyro_x,gyro_y,gyro_z
  Frame Transfer : Subsystem
  Frame Transfer1 : Subsystem
  Out1 : Outport
  wires:
  Frame Transfer1/3(Out3) -> Bus Creator/7  "gyro_z"
  Frame Transfer1/2(Out2) -> Bus Creator/6  "gyro_y"
  Frame Transfer1/1(Out1) -> Bus Creator/5  "gyro_x"
  Bus Selector/7 -> Frame Transfer1/3(In3)  "<gyro_z>"
  Bus Selector/6 -> Frame Transfer1/2(In2)  "<gyro_y>"
  Bus Selector/5 -> Frame Transfer1/1(In1)  "<gyro_x>"
  Frame Transfer/3(Out3) -> Bus Creator/4  "accel_z"
  Frame Transfer/2(Out2) -> Bus Creator/3  "accel_y"
  Frame Transfer/1(Out1) -> Bus Creator/2  "accel_x"
  Bus Selector/4 -> Frame Transfer/3(In3)  "<accel_z>"
  Bus Selector/3 -> Frame Transfer/2(In2)  "<accel_y>"
  Bus Selector/2 -> Frame Transfer/1(In1)  "<accel_x>"
  In1/1 -> Bus Selector/1
  Bus Creator/1 -> Out1/1
  Bus Selector/1 -> Bus Creator/1  "<time>"

== system model_V1000Sim/FlightControl/sensor data frame transfer/SensorFrame to BodyFrame2 ==
  In1 : Inport
  Bus Creator : BusCreator  Inputs=7
  Bus Selector : BusSelector  OutputSignals=time,accel_x,accel_y,accel_z,gyro_x,gyro_y,gyro_z
  Frame Transfer : Subsystem
  Frame Transfer1 : Subsystem
  Out1 : Outport
  wires:
  Bus Selector/1 -> Bus Creator/1  "<time>"
  Bus Creator/1 -> Out1/1
  In1/1 -> Bus Selector/1
  Bus Selector/2 -> Frame Transfer/1(In1)  "<accel_x>"
  Bus Selector/3 -> Frame Transfer/2(In2)  "<accel_y>"
  Bus Selector/4 -> Frame Transfer/3(In3)  "<accel_z>"
  Frame Transfer/1(Out1) -> Bus Creator/2  "accel_x"
  Frame Transfer/2(Out2) -> Bus Creator/3  "accel_y"
  Frame Transfer/3(Out3) -> Bus Creator/4  "accel_z"
  Bus Selector/5 -> Frame Transfer1/1(In1)  "<gyro_x>"
  Bus Selector/6 -> Frame Transfer1/2(In2)  "<gyro_y>"
  Bus Selector/7 -> Frame Transfer1/3(In3)  "<gyro_z>"
  Frame Transfer1/1(Out1) -> Bus Creator/5  "gyro_x"
  Frame Transfer1/2(Out2) -> Bus Creator/6  "gyro_y"
  Frame Transfer1/3(Out3) -> Bus Creator/7  "gyro_z"

== system model_V1000Sim/FlightControl/sensor data frame transfer/SensorFrame to BodyFrame3 ==
  In1 : Inport
  Bus Creator : BusCreator  Inputs=4
  Bus Selector : BusSelector  OutputSignals=time,mag_x,mag_y,mag_z
  Frame Transfer : Subsystem
  Out1 : Outport
  wires:
  Frame Transfer/3(Out3) -> Bus Creator/4  "mag_z"
  Frame Transfer/2(Out2) -> Bus Creator/3  "mag_y"
  Frame Transfer/1(Out1) -> Bus Creator/2  "mag_x"
  Bus Selector/4 -> Frame Transfer/3(In3)  "<mag_z>"
  Bus Selector/3 -> Frame Transfer/2(In2)  "<mag_y>"
  Bus Selector/2 -> Frame Transfer/1(In1)  "<mag_x>"
  In1/1 -> Bus Selector/1
  Bus Creator/1 -> Out1/1
  Bus Selector/1 -> Bus Creator/1  "<time>"

== system model_V1000Sim/FlightControl/sensor data frame transfer/SensorFrame to BodyFrame4 ==
  In1 : Inport
  Bus Creator : BusCreator  Inputs=4
  Bus Selector : BusSelector  OutputSignals=time,mag_x,mag_y,mag_z
  Frame Transfer : Subsystem
  Out1 : Outport
  wires:
  Bus Selector/1 -> Bus Creator/1  "<time>"
  Bus Creator/1 -> Out1/1
  In1/1 -> Bus Selector/1
  Bus Selector/2 -> Frame Transfer/1(In1)  "<mag_x>"
  Bus Selector/3 -> Frame Transfer/2(In2)  "<mag_y>"
  Bus Selector/4 -> Frame Transfer/3(In3)  "<mag_z>"
  Frame Transfer/1(Out1) -> Bus Creator/2  "mag_x"
  Frame Transfer/2(Out2) -> Bus Creator/3  "mag_y"
  Frame Transfer/3(Out3) -> Bus Creator/4  "mag_z"

== system model_V1000Sim/数据显示/Sim Data/Subsystem ==
  Inport : Inport
  Inport1 : Inport  Port=2
  Demux7 : Demux  Outputs=3
  Demux8 : Demux  Outputs=3
  Mux : Mux  Inputs=2
  Mux1 : Mux  Inputs=2
  Mux2 : Mux  Inputs=2
  Outport : Outport
  Outport1 : Outport  Port=2
  Outport2 : Outport  Port=3
  wires:
  Demux7/1 -> Mux/1  "yaw [deg]"
  Demux8/1 -> Mux/2  "yaw [deg]"
  Inport/1 -> Demux7/1
  Mux/1 -> Outport/1
  Demux8/3 -> Mux2/2  "roll [deg]"
  Demux7/2 -> Mux1/1
  Inport1/1 -> Demux8/1
  Mux2/1 -> Outport2/1
  Mux1/1 -> Outport1/1
  Demux8/2 -> Mux1/2  "pitch [deg]"
  Demux7/3 -> Mux2/1  "roll [deg]"

== system model_V1000Sim/数据显示/Sim Data/Subsystem1 ==
  Inport : Inport
  Inport1 : Inport  Port=2
  Enable : EnablePort
  Demux7 : Demux  Outputs=3
  Demux8 : Demux  Outputs=3
  Mux : Mux  Inputs=2
  Mux1 : Mux  Inputs=2
  Mux2 : Mux  Inputs=2
  lat : Outport
  lon : Outport  Port=2
  alt : Outport  Port=3
  wires:
  Demux7/3 -> Mux2/1  "roll [deg]"
  Demux8/2 -> Mux1/2  "pitch [deg]"
  Mux2/1 -> alt/1
  Inport1/1 -> Demux8/1
  Demux7/2 -> Mux1/1
  Demux8/3 -> Mux2/2  "roll [deg]"
  Inport/1 -> Demux7/1
  Demux8/1 -> Mux/2  "yaw [deg]"
  Demux7/1 -> Mux/1  "yaw [deg]"
  Mux/1 -> lat/1
  Mux1/1 -> lon/1

== system model_V1000Sim/数据显示/Sim Data/Subsystem2 ==
  Inport : Inport
  Inport1 : Inport  Port=2
  Demux7 : Demux  Outputs=3
  Demux8 : Demux  Outputs=3
  Mux : Mux  Inputs=2
  Mux1 : Mux  Inputs=2
  Mux2 : Mux  Inputs=2
  Outport : Outport
  Outport1 : Outport  Port=2
  Outport2 : Outport  Port=3
  wires:
  Demux7/1 -> Mux/1  "yaw [deg]"
  Demux8/1 -> Mux/2  "yaw [deg]"
  Inport/1 -> Demux7/1
  Mux/1 -> Outport/1
  Demux8/3 -> Mux2/2  "roll [deg]"
  Demux7/2 -> Mux1/1
  Inport1/1 -> Demux8/1
  Mux2/1 -> Outport2/1
  Mux1/1 -> Outport1/1
  Demux8/2 -> Mux1/2  "pitch [deg]"
  Demux7/3 -> Mux2/1  "roll [deg]"

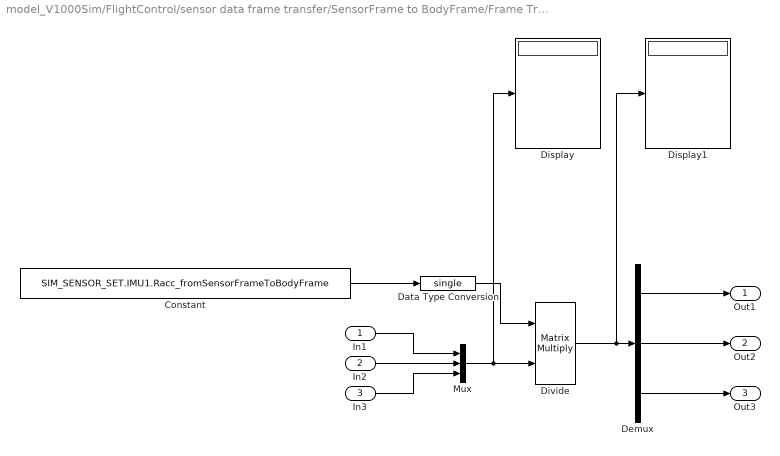
== system model_V1000Sim/FlightControl/sensor data frame transfer/SensorFrame to BodyFrame/Frame Transfer ==
  In1 : Inport
  In2 : Inport  Port=2
  In3 : Inport  Port=3
  Constant : Constant  Value=SIM_SENSOR_SET.IMU1.Racc_fromSensorFrameToBodyFrame
  Data Type Conversion : DataTypeConversion  OutDataTypeStr=single
  Demux : Demux  Outputs=3
  Display : Display
  Display1 : Display
  Divide : Product  Inputs=**  Multiplication=Matrix(*)
  Mux : Mux  Inputs=3
  Out1 : Outport
  Out2 : Outport  Port=2
  Out3 : Outport  Port=3
  wires:
  In2/1 -> Mux/2
  In1/1 -> Mux/1
  In3/1 -> Mux/3
  Constant/1 -> Data Type Conversion/1
  Mux/1 -> Display/1, Divide/2
  Divide/1 -> Display1/1, Demux/1
  Demux/1 -> Out1/1
  Demux/2 -> Out2/1
  Demux/3 -> Out3/1
  Data Type Conversion/1 -> Divide/1

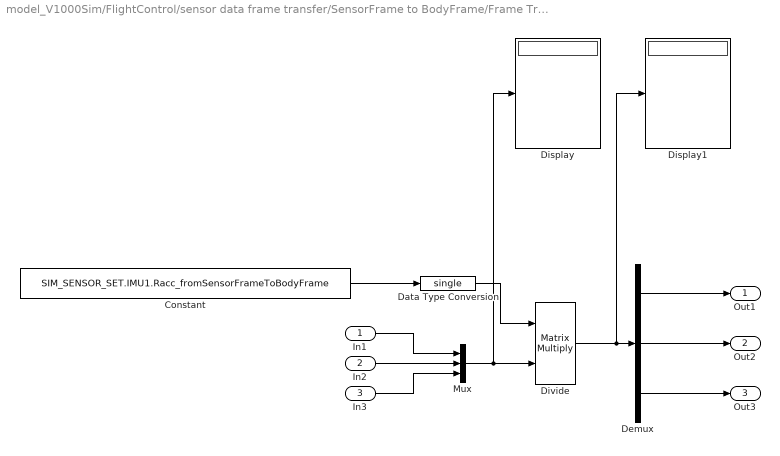
== system model_V1000Sim/FlightControl/sensor data frame transfer/SensorFrame to BodyFrame/Frame Transfer1 ==
  In1 : Inport
  In2 : Inport  Port=2
  In3 : Inport  Port=3
  Constant : Constant  Value=SIM_SENSOR_SET.IMU1.Racc_fromSensorFrameToBodyFrame
  Data Type Conversion : DataTypeConversion  OutDataTypeStr=single
  Demux : Demux  Outputs=3
  Display : Display
  Display1 : Display
  Divide : Product  Inputs=**  Multiplication=Matrix(*)
  Mux : Mux  Inputs=3
  Out1 : Outport
  Out2 : Outport  Port=2
  Out3 : Outport  Port=3
  wires:
  Data Type Conversion/1 -> Divide/1
  Demux/3 -> Out3/1
  Demux/2 -> Out2/1
  Demux/1 -> Out1/1
  Divide/1 -> Demux/1, Display1/1
  Mux/1 -> Divide/2, Display/1
  Constant/1 -> Data Type Conversion/1
  In3/1 -> Mux/3
  In1/1 -> Mux/1
  In2/1 -> Mux/2

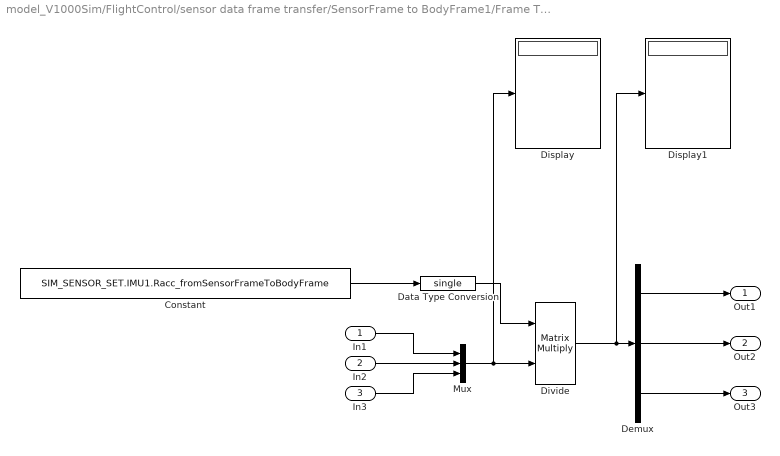
== system model_V1000Sim/FlightControl/sensor data frame transfer/SensorFrame to BodyFrame1/Frame Transfer ==
  In1 : Inport
  In2 : Inport  Port=2
  In3 : Inport  Port=3
  Constant : Constant  Value=SIM_SENSOR_SET.IMU1.Racc_fromSensorFrameToBodyFrame
  Data Type Conversion : DataTypeConversion  OutDataTypeStr=single
  Demux : Demux  Outputs=3
  Display : Display
  Display1 : Display
  Divide : Product  Inputs=**  Multiplication=Matrix(*)
  Mux : Mux  Inputs=3
  Out1 : Outport
  Out2 : Outport  Port=2
  Out3 : Outport  Port=3
  wires:
  Data Type Conversion/1 -> Divide/1
  Demux/3 -> Out3/1
  Demux/2 -> Out2/1
  Demux/1 -> Out1/1
  Divide/1 -> Demux/1, Display1/1
  Mux/1 -> Divide/2, Display/1
  Constant/1 -> Data Type Conversion/1
  In3/1 -> Mux/3
  In1/1 -> Mux/1
  In2/1 -> Mux/2

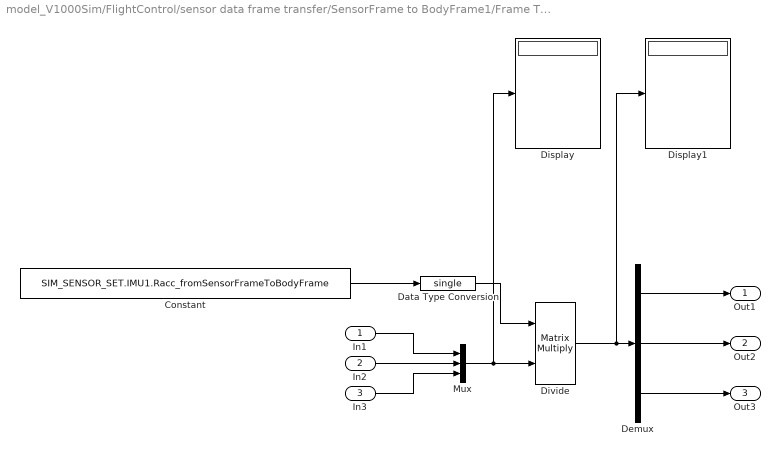
== system model_V1000Sim/FlightControl/sensor data frame transfer/SensorFrame to BodyFrame1/Frame Transfer1 ==
  In1 : Inport
  In2 : Inport  Port=2
  In3 : Inport  Port=3
  Constant : Constant  Value=SIM_SENSOR_SET.IMU1.Racc_fromSensorFrameToBodyFrame
  Data Type Conversion : DataTypeConversion  OutDataTypeStr=single
  Demux : Demux  Outputs=3
  Display : Display
  Display1 : Display
  Divide : Product  Inputs=**  Multiplication=Matrix(*)
  Mux : Mux  Inputs=3
  Out1 : Outport
  Out2 : Outport  Port=2
  Out3 : Outport  Port=3
  wires:
  In2/1 -> Mux/2
  In1/1 -> Mux/1
  In3/1 -> Mux/3
  Constant/1 -> Data Type Conversion/1
  Mux/1 -> Display/1, Divide/2
  Divide/1 -> Display1/1, Demux/1
  Demux/1 -> Out1/1
  Demux/2 -> Out2/1
  Demux/3 -> Out3/1
  Data Type Conversion/1 -> Divide/1

== system model_V1000Sim/FlightControl/sensor data frame transfer/SensorFrame to BodyFrame2/Frame Transfer ==
  In1 : Inport
  In2 : Inport  Port=2
  In3 : Inport  Port=3
  Constant : Constant  Value=SIM_SENSOR_SET.IMU1.Racc_fromSensorFrameToBodyFrame
  Data Type Conversion : DataTypeConversion  OutDataTypeStr=single
  Demux : Demux  Outputs=3
  Display : Display
  Display1 : Display
  Divide : Product  Inputs=**  Multiplication=Matrix(*)
  Mux : Mux  Inputs=3
  Out1 : Outport
  Out2 : Outport  Port=2
  Out3 : Outport  Port=3
  wires:
  In2/1 -> Mux/2
  In1/1 -> Mux/1
  In3/1 -> Mux/3
  Constant/1 -> Data Type Conversion/1
  Mux/1 -> Display/1, Divide/2
  Divide/1 -> Display1/1, Demux/1
  Demux/1 -> Out1/1
  Demux/2 -> Out2/1
  Demux/3 -> Out3/1
  Data Type Conversion/1 -> Divide/1

== system model_V1000Sim/FlightControl/sensor data frame transfer/SensorFrame to BodyFrame2/Frame Transfer1 ==
  In1 : Inport
  In2 : Inport  Port=2
  In3 : Inport  Port=3
  Constant : Constant  Value=SIM_SENSOR_SET.IMU1.Racc_fromSensorFrameToBodyFrame
  Data Type Conversion : DataTypeConversion  OutDataTypeStr=single
  Demux : Demux  Outputs=3
  Display : Display
  Display1 : Display
  Divide : Product  Inputs=**  Multiplication=Matrix(*)
  Mux : Mux  Inputs=3
  Out1 : Outport
  Out2 : Outport  Port=2
  Out3 : Outport  Port=3
  wires:
  Data Type Conversion/1 -> Divide/1
  Demux/3 -> Out3/1
  Demux/2 -> Out2/1
  Demux/1 -> Out1/1
  Divide/1 -> Demux/1, Display1/1
  Mux/1 -> Divide/2, Display/1
  Constant/1 -> Data Type Conversion/1
  In3/1 -> Mux/3
  In1/1 -> Mux/1
  In2/1 -> Mux/2

== system model_V1000Sim/FlightControl/sensor data frame transfer/SensorFrame to BodyFrame3/Frame Transfer ==
  In1 : Inport
  In2 : Inport  Port=2
  In3 : Inport  Port=3
  Constant : Constant  Value=SIM_SENSOR_SET.Mag1.R_fromSensorFrameToBodyFrame
  Data Type Conversion : DataTypeConversion  OutDataTypeStr=single
  Demux : Demux  Outputs=3
  Display : Display
  Display1 : Display
  Divide : Product  Inputs=**  Multiplication=Matrix(*)
  Mux : Mux  Inputs=3
  Out1 : Outport
  Out2 : Outport  Port=2
  Out3 : Outport  Port=3
  wires:
  Data Type Conversion/1 -> Divide/1
  Demux/3 -> Out3/1
  Demux/2 -> Out2/1
  Demux/1 -> Out1/1
  Divide/1 -> Demux/1, Display1/1
  Mux/1 -> Divide/2, Display/1
  Constant/1 -> Data Type Conversion/1
  In3/1 -> Mux/3
  In1/1 -> Mux/1
  In2/1 -> Mux/2

== system model_V1000Sim/FlightControl/sensor data frame transfer/SensorFrame to BodyFrame4/Frame Transfer ==
  In1 : Inport
  In2 : Inport  Port=2
  In3 : Inport  Port=3
  Constant : Constant  Value=SIM_SENSOR_SET.Mag2.R_fromSensorFrameToBodyFrame
  Data Type Conversion : DataTypeConversion  OutDataTypeStr=single
  Demux : Demux  Outputs=3
  Display : Display
  Display1 : Display
  Divide : Product  Inputs=**  Multiplication=Matrix(*)
  Mux : Mux  Inputs=3
  Out1 : Outport
  Out2 : Outport  Port=2
  Out3 : Outport  Port=3
  wires:
  In2/1 -> Mux/2
  In1/1 -> Mux/1
  In3/1 -> Mux/3
  Constant/1 -> Data Type Conversion/1
  Mux/1 -> Display/1, Divide/2
  Divide/1 -> Display1/1, Demux/1
  Demux/1 -> Out1/1
  Demux/2 -> Out2/1
  Demux/3 -> Out3/1
  Data Type Conversion/1 -> Divide/1
